simulink model "Speed_Dependant_Saturation"  (R2022a)
settings: Solver=VariableStepAuto  StartTime=0.0  StopTime=10  RelTol=1e-3
libraries: simulink x1
settings Model: Creator=maxju  LastModifiedBy=maxju

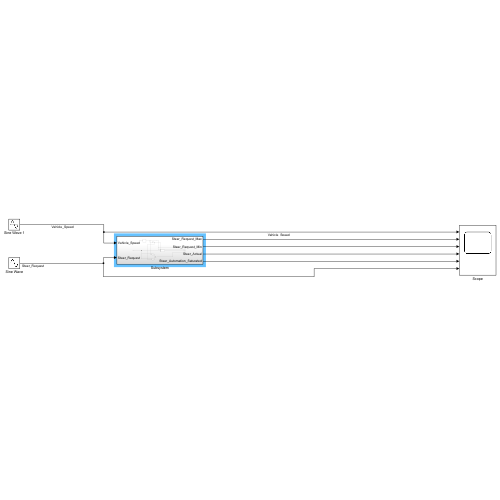
[thumbnail: Simulink's stored preview of the top-level diagram]
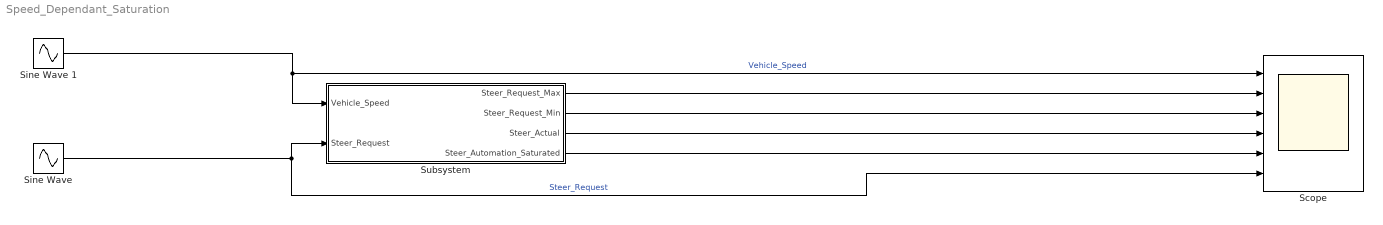
== system Speed_Dependant_Saturation ==
  Scope : Scope  NumInputPorts=6
  Sine Wave : Sin  Amplitude=100  SampleTime=0
  Sine Wave 1 : Sin  Amplitude=50  Bias=50  SampleTime=0
  Subsystem : Subsystem
  wires:
  Sine Wave 1/1 -> Subsystem/1(Vehicle_Speed), Scope/1  "Vehicle_Speed"
  Sine Wave/1 -> Subsystem/2(Steer_Request), Scope/6  "Steer_Request"
  Subsystem/1(Steer_Request_Max) -> Scope/2
  Subsystem/2(Steer_Request_Min) -> Scope/3
  Subsystem/3(Steer_Actual) -> Scope/4
  Subsystem/4(Steer_Automation_Saturated) -> Scope/5

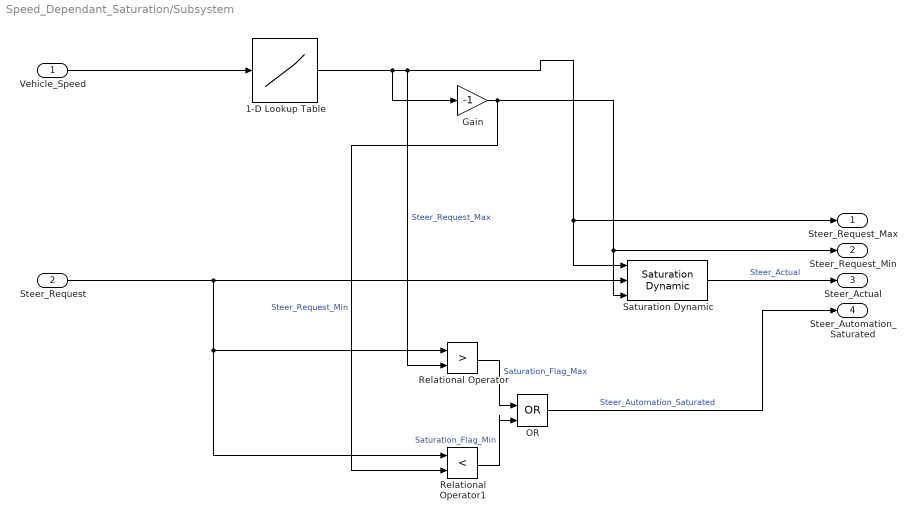
== system Speed_Dependant_Saturation/Subsystem ==
  Vehicle_Speed : Inport
  Steer_Request : Inport  Port=2
  1-D Lookup Table : Lookup_n-D  NumberOfTableDimensions=1  BreakpointsForDimension1=[0,10,20,30,50]  Table=[100,100,60,40,30]  InternalRulePriority=Speed  RndMeth=Simplest
  Gain : Gain  Gain=-1
  OR : Logic  Operator=OR  IconShape=distinctive  AllPortsSameDT=off  OutDataTypeStr=boolean
  Relational Operator : RelationalOperator  Operator=>  OutDataTypeStr=boolean  RndMeth=Simplest  InputSameDT=off
  Relational Operator1 : RelationalOperator  Operator=<  OutDataTypeStr=boolean  RndMeth=Simplest  InputSameDT=off
  Saturation Dynamic : simulink/Discontinuities/Saturation Dynamic  OutMin=[]  OutMax=[]  OutDataTypeStr=Inherit: Same as second input  OutDataType=fixdt(1, 16)  OutScaling=2^-10  DoSatur=off
  Steer_Request_Max : Outport
  Steer_Request_Min : Outport  Port=2
  Steer_Actual : Outport  Port=3
  Steer_Automation_Saturated : Outport  Port=4
  wires:
  1-D Lookup Table/1 -> Relational Operator/2, Steer_Request_Max/1, Saturation Dynamic/1, Gain/1  "Steer_Request_Max"
  OR/1 -> Steer_Automation_Saturated/1  "Steer_Automation_Saturated"
  Relational Operator1/1 -> OR/2  "Saturation_Flag_Min"
  Relational Operator/1 -> OR/1  "Saturation_Flag_Max"
  Steer_Request/1 -> Saturation Dynamic/2, Relational Operator1/1, Relational Operator/1
  Gain/1 -> Relational Operator1/2, Steer_Request_Min/1, Saturation Dynamic/3  "Steer_Request_Min"
  Vehicle_Speed/1 -> 1-D Lookup Table/1
  Saturation Dynamic/1 -> Steer_Actual/1  "Steer_Actual"
